simulink model "lagrange_model_v2"  (R2022a)
settings: Solver=VariableStepAuto  StartTime=0.0  StopTime=10.0  RelTol=1e-3
(part 1 of 3)
settings Model: Creator=legacy  LastModifiedBy=legacy

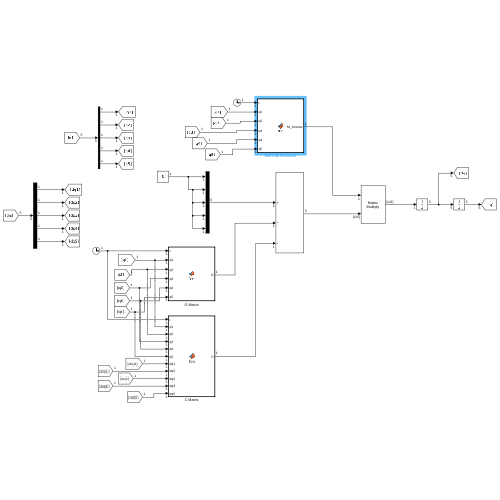
[thumbnail: Simulink's stored preview of the top-level diagram]
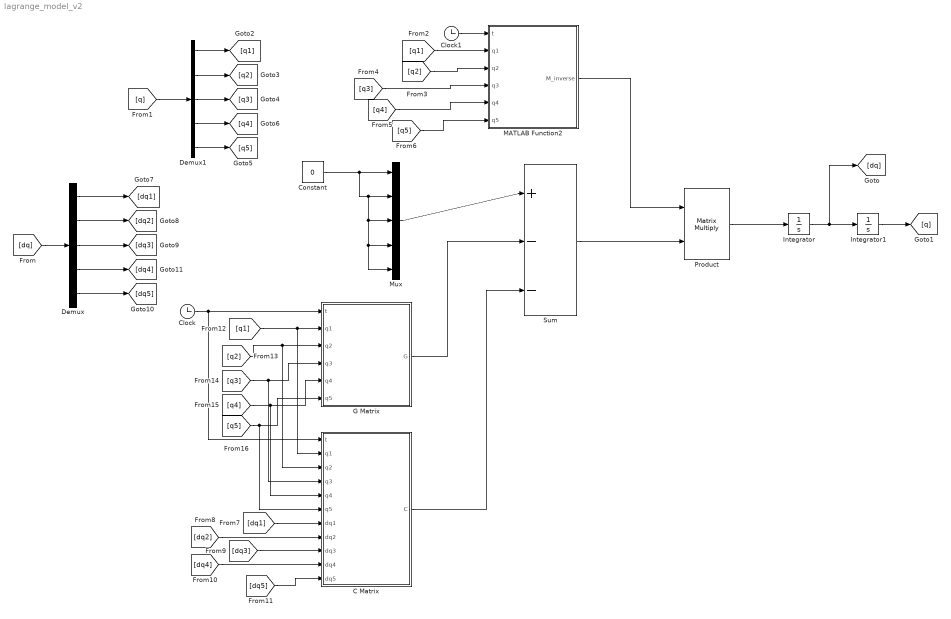
== system lagrange_model_v2 ==
  C Matrix : MATLAB Function  TreatAsAtomicUnit=on
  Clock : Clock
  Clock1 : Clock
  Constant : Constant  Value=0
  Demux : Demux  Outputs=5
  Demux1 : Demux  Outputs=5
  G Matrix : MATLAB Function  TreatAsAtomicUnit=on
  Integrator : Integrator  InitialCondition=[0, 0, 0, 0, 0]
  Integrator1 : Integrator  InitialCondition=[0, 0, 0, 0, 0]
  MATLAB Function2 : MATLAB Function  TreatAsAtomicUnit=on
  Mux : Mux  Inputs=5
  Product : Product  Multiplication=Matrix(*)
  Sum : Sum  Inputs=|+--
  wires:
  Clock/1 -> C Matrix/1(t), G Matrix/1(t)
  Constant/1 -> Mux/5, Mux/4, Mux/3, Mux/2, Mux/1
  Mux/1 -> Sum/1
  G Matrix/1(G) -> Sum/2
  C Matrix/1(C) -> Sum/3
  Sum/1 -> Product/2
  Clock1/1 -> MATLAB Function2/1(t)
  MATLAB Function2/1(M_inverse) -> Product/1
  Product/1 -> Integrator/1
  Integrator/1 -> [dq], Integrator1/1
  Integrator1/1 -> [q]
  [q] -> Demux1/1
  Demux1/1 -> [q1]
  Demux1/2 -> [q2]
  Demux1/3 -> [q3]
  Demux1/4 -> [q4]
  Demux1/5 -> [q5]
  [q1] -> MATLAB Function2/2(q1)
  [q2] -> MATLAB Function2/3(q2)
  [q3] -> MATLAB Function2/4(q3)
  [q4] -> MATLAB Function2/5(q4)
  [q5] -> MATLAB Function2/6(q5)
  [dq] -> Demux/1
  Demux/1 -> [dq1]
  Demux/2 -> [dq2]
  Demux/3 -> [dq3]
  Demux/4 -> [dq4]
  Demux/5 -> [dq5]
  [dq1] -> C Matrix/7(dq1)
  [dq2] -> C Matrix/8(dq2)
  [dq3] -> C Matrix/9(dq3)
  [dq4] -> C Matrix/10(dq4)
  [dq5] -> C Matrix/11(dq5)
  [q1] -> C Matrix/2(q1), G Matrix/2(q1)
  [q2] -> C Matrix/3(q2), G Matrix/3(q2)
  [q3] -> C Matrix/4(q3), G Matrix/4(q3)
  [q4] -> C Matrix/5(q4), G Matrix/5(q4)
  [q5] -> C Matrix/6(q5), G Matrix/6(q5)

== matlab function lagrange_model_v2/C Matrix ==
  data: t input; q1 input; C output; q2 input; q3 input; q4 input; q5 input; dq1 input; dq2 input; dq3 input; dq4 input; dq5 input
function C = fcn(t, q1, q2, q3, q4, q5, dq1, dq2, dq3, dq4, dq5)


lb1 = 0.025; l1 = 0.110; l2 = 0.38; l3 = 0.38, l4 = 0.38; l5 = 0.04;
pi = 3.14159; beta1 = 0.3; beta2 = 0.1; beta3 = 0.1; beta4 = 0.1; beta5 = 0.1;
g = 9.81; 
m1 = 2.24036; m2 = 1.380584; m3 = 0.4927734;
m4 = 1.380584; m5 = 0.130378439395373;
% Inertia Tensor 1:
Ixx1 = 0.00602313752636761; Ixy1 = 2.1208125474502E-05; Ixz1 = 0;
Iyx1 = -Ixy1; Iyy1 = 0.00579248437417585; Iyz1 = 0;
Izx1 = -Ixz1; Izy1 = -Iyz1; Izz1 = 0.0098329939500295;

% Inertia Tensor 2:
Ixx2 = 0.00248849839; Ixy2 = 0; Ixz2 = 0;
Iyx2 = -Ixy2; Iyy2 = 0.043747624; Iyz2 = 0;
Izx2 = -Ixz2; Izy2 = -Iyz2; Izz = 0.0425687;

% Intertia Tensor 3:
Ixx3 = 0.000993126; Ixy3 = 0; Ixz3 = 0;
Iyx3 = -Ixy3; Iyy3 = 0.0088282898; Iyz3 = 0;
Izx3 = -Ixz3; Izy3 = -Iyz3; Izz3 = 0.008576398866;

% Intertia Tensor 4:
Ixx4 = 0.00312638; Ixy4 = 0.00354785; Ixz4 = 0.0035964956;
Iyx4 = -Ixy4; Iyy4 = 0.0434376808; Iyz4 = -0.00032350627;
Izx4 = -Ixz4; Izy4 = -Iyz4; Izz4 = 0.042240781;

% Intertia Tensor 5:
Ixx5 = 9.85693744749924E-05; Ixy5 = 0; Ixz5 = 0;
Iyx5 = -Ixy5; Iyy5 = 0.00011697309; Iyz5 = 0;
Izx5 = -Ixz5; Izy5 = -Iyz5; Izz5 = 0.0001866513337855;

C = evalin('base', 'C_matrix_t');

== matlab function lagrange_model_v2/G Matrix ==
  data: t input; q1 input; G output; q2 input; q3 input; q4 input; q5 input
function G = fcn(t, q1, q2, q3, q4, q5)


lb1 = 0.025; l1 = 0.110; l2 = 0.38; l3 = 0.38, l4 = 0.38; l5 = 0.04;
pi = 3.14159; beta1 = 0.3; beta2 = 0.1; beta3 = 0.1; beta4 = 0.1; beta5 = 0.1;
g = 9.81; 
m1 = 2.24036; m2 = 1.380584; m3 = 0.4927734;
m4 = 1.380584; m5 = 0.130378439395373;
% Inertia Tensor 1:
Ixx1 = 0.00602313752636761; Ixy1 = 2.1208125474502E-05; Ixz1 = 0;
Iyx1 = -Ixy1; Iyy1 = 0.00579248437417585; Iyz1 = 0;
Izx1 = -Ixz1; Izy1 = -Iyz1; Izz1 = 0.0098329939500295;

% Inertia Tensor 2:
Ixx2 = 0.00248849839; Ixy2 = 0; Ixz2 = 0;
Iyx2 = -Ixy2; Iyy2 = 0.043747624; Iyz2 = 0;
Izx2 = -Ixz2; Izy2 = -Iyz2; Izz = 0.0425687;

% Intertia Tensor 3:
Ixx3 = 0.000993126; Ixy3 = 0; Ixz3 = 0;
Iyx3 = -Ixy3; Iyy3 = 0.0088282898; Iyz3 = 0;
Izx3 = -Ixz3; Izy3 = -Iyz3; Izz3 = 0.008576398866;

% Intertia Tensor 4:
Ixx4 = 0.00312638; Ixy4 = 0.00354785; Ixz4 = 0.0035964956;
Iyx4 = -Ixy4; Iyy4 = 0.0434376808; Iyz4 = -0.00032350627;
Izx4 = -Ixz4; Izy4 = -Iyz4; Izz4 = 0.042240781;

% Intertia Tensor 5:
Ixx5 = 9.85693744749924E-05; Ixy5 = 0; Ixz5 = 0;
Iyx5 = -Ixy5; Iyy5 = 0.00011697309; Iyz5 = 0;
Izx5 = -Ixz5; Izy5 = -Iyz5; Izz5 = 0.0001866513337855;

G11 = 0;
G12 = 3.5358e-11*sin(th2(t)) - 10.043*cos(th2(t)) + 6.551*sin(th3(t))*(3.5208e-12*cos(th2(t) - 1.5708) + 1.0*sin(th2(t) - 1.5708)) - 0.02558*sin(th5(t))*(cos(th4(t) - 3.1416)*(cos(th3(t) - 1.5708)*(3.5208e-12*cos(th2(t) - 1.5708) + 1.0*sin(th2(t) - 1.5708)) + sin(th3(t) - 1.5708)*(1.0*cos(th2(t) - 1.5708) - 3.5208e-12*sin(th2(t) - 1.5708))) - 1.0*sin(th4(t) - 3.1416)*(cos(th3(t) - 1.5708)*(1.0*cos(th2(t) - 1.5708) - 3.5208e-12*sin(th2(t) - 1.5708)) - 1.0*sin(th3(t) - 1.5708)*(3.5208e-12*cos(th2(t) - 1.5708) + 1.0*sin(th2(t) - 1.5708)))) + 3.0593*sin(th4(t))*(cos(th3(t) - 1.5708)*(3.5208e-12*cos(th2(t) - 1.5708) + 1.0*sin(th2(t) - 1.5708)) + sin(th3(t) - 1.5708)*(1.0*cos(th2(t) - 1.5708) - 3.5208e-12*sin(th2(t) - 1.5708))) - 3.0593*cos(th4(t))*(cos(th3(t) - 1.5708)*(1.0*cos(th2(t) - 1.5708) - 3.5208e-12*sin(th2(t) - 1.5708)) - 1.0*sin(th3(t) - 1.5708)*(3.5208e-12*cos(th2(t) - 1.5708) + 1.0*sin(th2(t) - 1.5708))) - 6.551*cos(th3(t))*(1.0*cos(th2(t) - 1.5708) - 3.5208e-12*sin(th2(t) - 1.5708)) + 0.02558*cos(th5(t))*(sin(th4(t) - 3.1416)*(cos(th3(t) - 1.5708)*(3.5208e-12*cos(th2(t) - 1.5708) + 1.0*sin(th2(t) - 1.5708)) + sin(th3(t) - 1.5708)*(1.0*cos(th2(t) - 1.5708) - 3.5208e-12*sin(th2(t) - 1.5708))) + cos(th4(t) - 3.1416)*(cos(th3(t) - 1.5708)*(1.0*cos(th2(t) - 1.5708) - 3.5208e-12*sin(th2(t) - 1.5708)) - 1.0*sin(th3(t) - 1.5708)*(3.5208e-12*cos(th2(t) - 1.5708) + 1.0*sin(th2(t) - 1.5708))));
G13 = 6.551*sin(th3(t))*(3.5208e-12*cos(th2(t) - 1.5708) + 1.0*sin(th2(t) - 1.5708)) - 0.02558*sin(th5(t))*(cos(th4(t) - 3.1416)*(cos(th3(t) - 1.5708)*(3.5208e-12*cos(th2(t) - 1.5708) + 1.0*sin(th2(t) - 1.5708)) + sin(th3(t) - 1.5708)*(1.0*cos(th2(t) - 1.5708) - 3.5208e-12*sin(th2(t) - 1.5708))) - 1.0*sin(th4(t) - 3.1416)*(cos(th3(t) - 1.5708)*(1.0*cos(th2(t) - 1.5708) - 3.5208e-12*sin(th2(t) - 1.5708)) - 1.0*sin(th3(t) - 1.5708)*(3.5208e-12*cos(th2(t) - 1.5708) + 1.0*sin(th2(t) - 1.5708)))) + 3.0593*sin(th4(t))*(cos(th3(t) - 1.5708)*(3.5208e-12*cos(th2(t) - 1.5708) + 1.0*sin(th2(t) - 1.5708)) + sin(th3(t) - 1.5708)*(1.0*cos(th2(t) - 1.5708) - 3.5208e-12*sin(th2(t) - 1.5708))) - 3.0593*cos(th4(t))*(cos(th3(t) - 1.5708)*(1.0*cos(th2(t) - 1.5708) - 3.5208e-12*sin(th2(t) - 1.5708)) - 1.0*sin(th3(t) - 1.5708)*(3.5208e-12*cos(th2(t) - 1.5708) + 1.0*sin(th2(t) - 1.5708))) - 6.551*cos(th3(t))*(1.0*cos(th2(t) - 1.5708) - 3.5208e-12*sin(th2(t) - 1.5708)) + 0.02558*cos(th5(t))*(sin(th4(t) - 3.1416)*(cos(th3(t) - 1.5708)*(3.5208e-12*cos(th2(t) - 1.5708) + 1.0*sin(th2(t) - 1.5708)) + sin(th3(t) - 1.5708)*(1.0*cos(th2(t) - 1.5708) - 3.5208e-12*sin(th2(t) - 1.5708))) + cos(th4(t) - 3.1416)*(cos(th3(t) - 1.5708)*(1.0*cos(th2(t) - 1.5708) - 3.5208e-12*sin(th2(t) - 1.5708)) - 1.0*sin(th3(t) - 1.5708)*(3.5208e-12*cos(th2(t) - 1.5708) + 1.0*sin(th2(t) - 1.5708))));
G14 = 0.02558*sin(th5(t))*(cos(th4(t) - 3.1416)*(cos(th3(t) - 1.5708)*(3.5208e-12*cos(th2(t) - 1.5708) + 1.0*sin(th2(t) - 1.5708)) + sin(th3(t) - 1.5708)*(1.0*cos(th2(t) - 1.5708) - 3.5208e-12*sin(th2(t) - 1.5708))) - 1.0*sin(th4(t) - 3.1416)*(cos(th3(t) - 1.5708)*(1.0*cos(th2(t) - 1.5708) - 3.5208e-12*sin(th2(t) - 1.5708)) - 1.0*sin(th3(t) - 1.5708)*(3.5208e-12*cos(th2(t) - 1.5708) + 1.0*sin(th2(t) - 1.5708)))) + 3.0593*sin(th4(t))*(cos(th3(t) - 1.5708)*(3.5208e-12*cos(th2(t) - 1.5708) + 1.0*sin(th2(t) - 1.5708)) + sin(th3(t) - 1.5708)*(1.0*cos(th2(t) - 1.5708) - 3.5208e-12*sin(th2(t) - 1.5708))) - 3.0593*cos(th4(t))*(cos(th3(t) - 1.5708)*(1.0*cos(th2(t) - 1.5708) - 3.5208e-12*sin(th2(t) - 1.5708)) - 1.0*sin(th3(t) - 1.5708)*(3.5208e-12*cos(th2(t) - 1.5708) + 1.0*sin(th2(t) - 1.5708))) - 0.02558*cos(th5(t))*(sin(th4(t) - 3.1416)*(cos(th3(t) - 1.5708)*(3.5208e-12*cos(th2(t) - 1.5708) + 1.0*sin(th2(t) - 1.5708)) + sin(th3(t) - 1.5708)*(1.0*cos(th2(t) - 1.5708) - 3.5208e-12*sin(th2(t) - 1.5708))) + cos(th4(t) - 3.1416)*(cos(th3(t) - 1.5708)*(1.0*cos(th2(t) - 1.5708) - 3.5208e-12*sin(th2(t) - 1.5708)) - 1.0*sin(th3(t) - 1.5708)*(3.5208e-12*cos(th2(t) - 1.5708) + 1.0*sin(th2(t) - 1.5708))));
G15 = 0.02558*cos(th5(t))*(sin(th4(t) - 3.1416)*(cos(th3(t) - 1.5708)*(3.5208e-12*cos(th2(t) - 1.5708) + 1.0*sin(th2(t) - 1.5708)) + sin(th3(t) - 1.5708)*(1.0*cos(th2(t) - 1.5708) - 3.5208e-12*sin(th2(t) - 1.5708))) + cos(th4(t) - 3.1416)*(cos(th3(t) - 1.5708)*(1.0*cos(th2(t) - 1.5708) - 3.5208e-12*sin(th2(t) - 1.5708)) - 1.0*sin(th3(t) - 1.5708)*(3.5208e-12*cos(th2(t) - 1.5708) + 1.0*sin(th2(t) - 1.5708)))) - 0.02558*sin(th5(t))*(cos(th4(t) - 3.1416)*(cos(th3(t) - 1.5708)*(3.5208e-12*cos(th2(t) - 1.5708) + 1.0*sin(th2(t) - 1.5708)) + sin(th3(t) - 1.5708)*(1.0*cos(th2(t) - 1.5708) - 3.5208e-12*sin(th2(t) - 1.5708))) - 1.0*sin(th4(t) - 3.1416)*(cos(th3(t) - 1.5708)*(1.0*cos(th2(t) - 1.5708) - 3.5208e-12*sin(th2(t) - 1.5708)) - 1.0*sin(th3(t) - 1.5708)*(3.5208e-12*cos(th2(t) - 1.5708) + 1.0*sin(th2(t) - 1.5708))));

G = [G11; G12; G13; G14; G15];
